simulink model "motorRegulator"  (R2018a)
settings: Solver=ode45  StartTime=0.0  StopTime=5  RelTol=1e-3  EnableMultiTasking=on
values from neighbouring files (symbols this model uses):
  A = [0 1 ... (first row only)    [servo.m]    (also in trains.m = [0 1 0 0; useGainsTrains.m = [0 1 0 0)
  B = [0; beta]    [servo.m]    (also in trains.m = [0; 0; 0; 1/M2]; useGainsTrains.m = [0; 0; 0; 1/M2])
  C = [1 0]    [servo.m]    (also in trains.m = [1 0 0 0]; useGainsTrains.m = [1 0 -1 0])
  K = [c*q1, (1/beta)*(sqrt(alpha^2+2*q1*beta*c)-alpha)]    [servo.m]    (also in useGainsTrains.m = inv(R) * B' * MHat)
settings Model: Creator=rae  LastModifiedBy=mqm
settings DataIOCC: LimitDataPoints=on  SaveFormat=Array
settings OptimizationCC: LifeSpan=inf
settings DebuggingCC: SFUnexpectedBacktrackingDiag=warning  SFNoUnconditionalDefaultTransitionDiag=warning  SFExecutionAtInitializationDiag=none
settings HardwareCC: ProdBitPerPointer=32  ProdBitPerSizeT=32  ProdBitPerPtrDiffT=32  ProdLargestAtomicFloat=None  ProdIntDivRoundTo=Undefined  ProdEndianess=Unspecified  ProdWordSize=32  ProdHWDeviceType=32-bit Generic
settings ModelReferenceCC: PropagateSignalLabelsOutOfModel=off
settings CodeAppCC: StateflowObjectComments=on
settings GRTTargetCC: TargetLangStandard=C89/C90 (ANSI)  GeneratePreprocessorConditionals=Disable all
settings ConfigComp: CovMetricSettings=dw  CovHtmlReporting=on  CovSaveCumulativeToWorkspaceVar=on  CovSaveSingleToWorkspaceVar=on  CovExternalEMLEnable=off

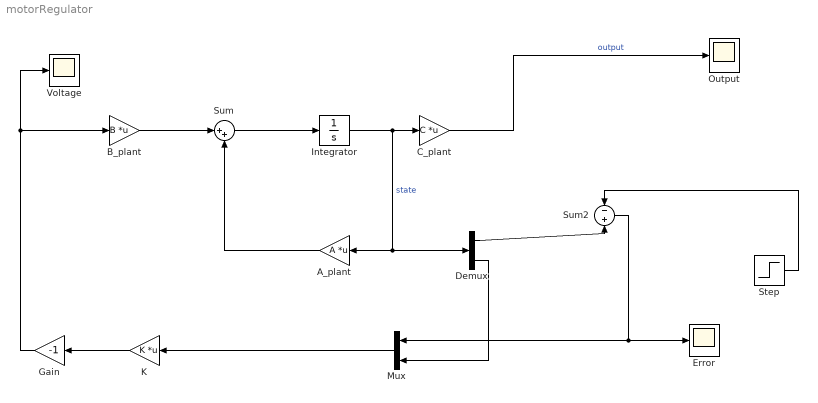
== system motorRegulator ==
  A_plant : Gain  Gain=A  Multiplication=Matrix(K*u)
  B_plant : Gain  Gain=B  Multiplication=Matrix(K*u)
  C_plant : Gain  Gain=C  Multiplication=Matrix(K*u)
  Demux : Demux  Outputs=2
  Error : Scope
  Gain : Gain  Gain=-1
  Integrator : Integrator
  K : Gain  Gain=K  Multiplication=Matrix(K*u)
  Mux : Mux  Inputs=2
  Output : Scope
  Step : Step  Time=0  SampleTime=0
  Sum : Sum  Inputs=|++
  Sum2 : Sum  Inputs=-+
  Voltage : Scope
  wires:
  B_plant/1 -> Sum/1
  Sum/1 -> Integrator/1
  Integrator/1 -> Demux/1, A_plant/1, C_plant/1  "state"
  A_plant/1 -> Sum/2
  C_plant/1 -> Output/1  "output"
  Step/1 -> Sum2/1
  Demux/1 -> Sum2/2
  Mux/1 -> K/1
  Demux/2 -> Mux/2
  Sum2/1 -> Error/1, Mux/1
  K/1 -> Gain/1
  Gain/1 -> Voltage/1, B_plant/1
